simulink model "avg_inflow"  (R2022b)
settings: Solver=FixedStepDiscrete  StartTime=0  StopTime=duration  FixedStep=sample_time  RelTol=1e-3
values from neighbouring files (symbols this model uses):
  ParInflow_TUM =     [avg_inflow_params.mat]
libraries: simulink x10, dspstat3 x10
settings Model: Creator=Carlo_TUM  LastModifiedBy=Carlo_TUM
settings DataIOCC: LoadExternalInput=on  ReturnWorkspaceOutputs=off  ReturnWorkspaceOutputsName=off
settings OptimizationCC: DefaultParameterBehavior=Inlined  EnhancedBackFolding=on  PassReuseOutputArgsAs=Individual arguments  OptimizeBlockOrder=speed  DifferentSizesBufferReuse=on  OptimizationCustomize=off  EfficientTunableParamExpr=on
settings DebuggingCC: ParameterTunabilityLossMsg=error
settings SFSimCC: MATLABDynamicMemAlloc=off
settings RTWCC: Description=Embedded Coder  SystemTargetFile=ert.tlc  TemplateMakefile=ert_default_tmf
settings CodeAppCC: ForceParamTrailComments=on  IgnoreCustomStorageClasses=off  OperatorAnnotations=on  SimulinkDataObjDesc=on  SFDataObjDesc=on  InsertBlockDesc=on
settings ERTTargetCC: TargetLangStandard=C99 (ISO)  GenerateSampleERTMain=on  InlinedParameterPlacement=NonHierarchical  ERTCustomFileTemplate=example_file_process.tlc

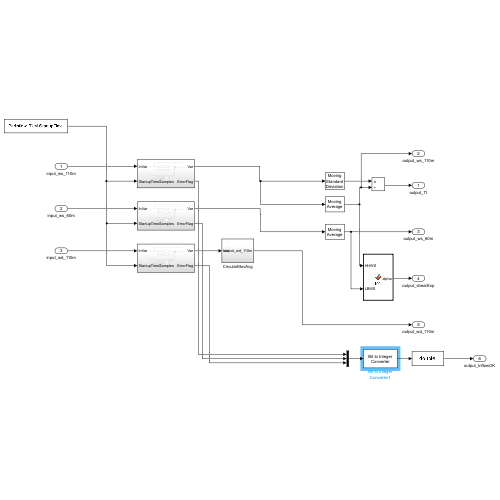
[thumbnail: Simulink's stored preview of the top-level diagram]
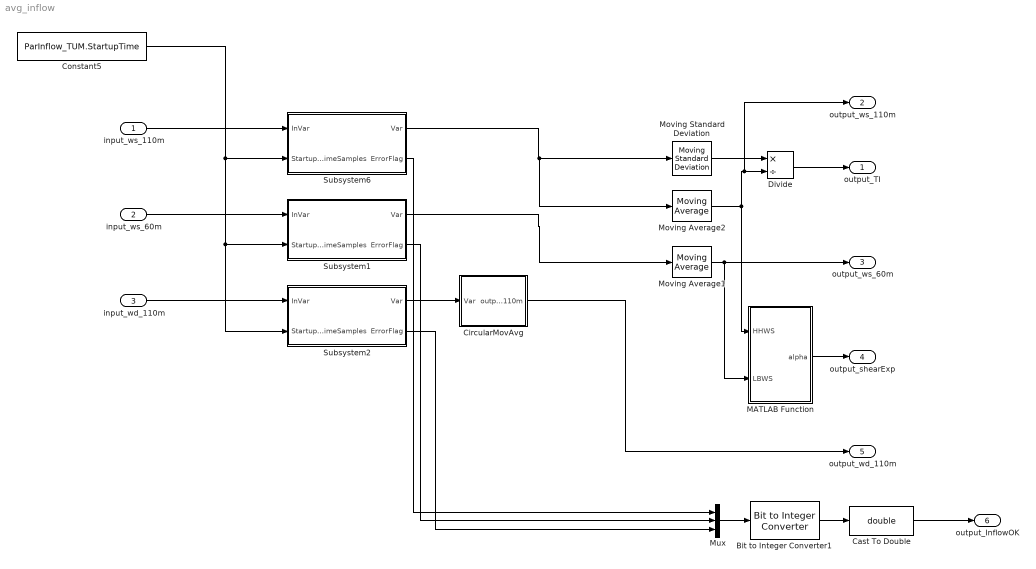
== system avg_inflow ==
  input_ws_110m : Inport  PortDimensions=1
  input_ws_60m : Inport  Port=2  PortDimensions=1
  input_wd_110m : Inport  Port=3  PortDimensions=1
  Bit to Integer Converter1 : simulink/Logic and Bit Operations/Bit to Integer Converter  nbits=3  bitOrder=MSB first  signedOutputValues=Unsigned  outDtype=Inherit via internal rule  outDtypeSigned=Inherit via internal rule
      settings: LibrarySourceBlock=|
      | commutil2/Bit to Integer
      | Converter
  Cast To Double : DataTypeConversion  OutDataTypeStr=double  SaturateOnIntegerOverflow=off  RndMeth=Floor
  CircularMovAvg : Subsystem
  Constant5 : Constant  Value=ParInflow_TUM.StartupTime
  Divide : Product  Inputs=*/
  MATLAB Function : MATLAB Function  TreatAsAtomicUnit=on
  Moving Average1 : dspstat3/Moving Average  Method=Sliding window  ForgettingFactorPort=off  SpecifyWindowLength=on  WindowLength=ParInflow_TUM.MovAvTI  OverlapLength=ParInflow_TUM.MovAvTI-1  AllowArbitraryInputLength=off  ForgettingFactor=0.9  SimulateUsing=Code generation
  Moving Average2 : dspstat3/Moving Average  Method=Sliding window  ForgettingFactorPort=off  SpecifyWindowLength=on  WindowLength=ParInflow_TUM.MovAvTI  OverlapLength=ParInflow_TUM.MovAvTI-1  AllowArbitraryInputLength=off  ForgettingFactor=0.9  SimulateUsing=Code generation
  Moving Standard Deviation : dspstat3/Moving Standard Deviation  Method=Sliding window  ForgettingFactorPort=off  SpecifyWindowLength=on  WindowLength=ParInflow_TUM.MovAvTI  OverlapLength=ParInflow_TUM.MovAvTI-1  AllowArbitraryInputLength=off  ForgettingFactor=0.9  SimulateUsing=Code generation
  Mux : Mux  Inputs=3
  Subsystem1 : Subsystem
  Subsystem2 : Subsystem
  Subsystem6 : Subsystem
  output_TI : Outport  VectorParamsAs1DForOutWhenUnconnected=off
  output_ws_110m : Outport  Port=2  VectorParamsAs1DForOutWhenUnconnected=off
  output_ws_60m : Outport  Port=3  VectorParamsAs1DForOutWhenUnconnected=off
  output_shearExp : Outport  Port=4  VectorParamsAs1DForOutWhenUnconnected=off
  output_wd_110m : Outport  Port=5  VectorParamsAs1DForOutWhenUnconnected=off
  output_InflowOK : Outport  Port=6  VectorParamsAs1DForOutWhenUnconnected=off
  wires:
  input_ws_110m/1 -> Subsystem6/1(InVar)
  input_ws_60m/1 -> Subsystem1/1(InVar)
  input_wd_110m/1 -> Subsystem2/1(InVar)
  Constant5/1 -> Subsystem2/2(StartupTimeSamples), Subsystem1/2(StartupTimeSamples), Subsystem6/2(StartupTimeSamples)
  Subsystem6/1(Var) -> Moving Average2/1, Moving Standard Deviation/1
  Subsystem1/1(Var) -> Moving Average1/1
  Moving Standard Deviation/1 -> Divide/1
  Moving Average2/1 -> MATLAB Function/1(HHWS), output_ws_110m/1, Divide/2
  Divide/1 -> output_TI/1
  Moving Average1/1 -> output_ws_60m/1, MATLAB Function/2(LBWS)
  MATLAB Function/1(alpha) -> output_shearExp/1
  Subsystem2/1(Var) -> CircularMovAvg/1(Var)
  CircularMovAvg/1(output_wd_110m) -> output_wd_110m/1
  Subsystem6/2(ErrorFlag) -> Mux/1
  Mux/1 -> Bit to Integer Converter1/1
  Subsystem2/2(ErrorFlag) -> Mux/3
  Subsystem1/2(ErrorFlag) -> Mux/2
  Bit to Integer Converter1/1 -> Cast To Double/1
  Cast To Double/1 -> output_InflowOK/1

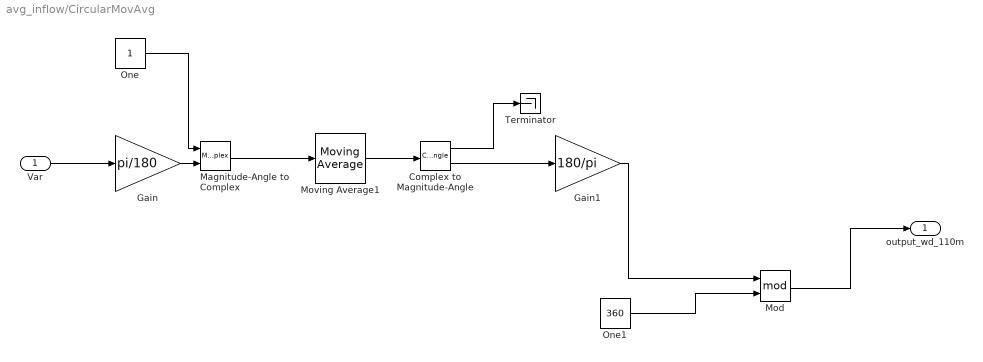
== system avg_inflow/CircularMovAvg ==
  Var : Inport
  Complex to Magnitude-Angle : ComplexToMagnitudeAngle
  Gain : Gain  Gain=pi/180
  Gain1 : Gain  Gain=180/pi
  Magnitude-Angle to Complex : MagnitudeAngleToComplex
  Mod : Math  Operator=mod  SignedPower=on
  Moving Average1 : dspstat3/Moving Average  Method=Sliding window  ForgettingFactorPort=off  SpecifyWindowLength=on  WindowLength=ParInflow_TUM.MovAvTI  OverlapLength=ParInflow_TUM.MovAvTI-1  AllowArbitraryInputLength=off  ForgettingFactor=0.9  SimulateUsing=Code generation
  One : Constant  OutDataTypeStr=Inherit: Inherit via back propagation
  One1 : Constant  Value=360  OutDataTypeStr=Inherit: Inherit via back propagation
  Terminator : Terminator
  output_wd_110m : Outport  VectorParamsAs1DForOutWhenUnconnected=off
  wires:
  Complex to Magnitude-Angle/2 -> Gain1/1
  Var/1 -> Gain/1
  One/1 -> Magnitude-Angle to Complex/1
  Gain/1 -> Magnitude-Angle to Complex/2
  Magnitude-Angle to Complex/1 -> Moving Average1/1
  Moving Average1/1 -> Complex to Magnitude-Angle/1
  Complex to Magnitude-Angle/1 -> Terminator/1
  Gain1/1 -> Mod/1
  One1/1 -> Mod/2
  Mod/1 -> output_wd_110m/1

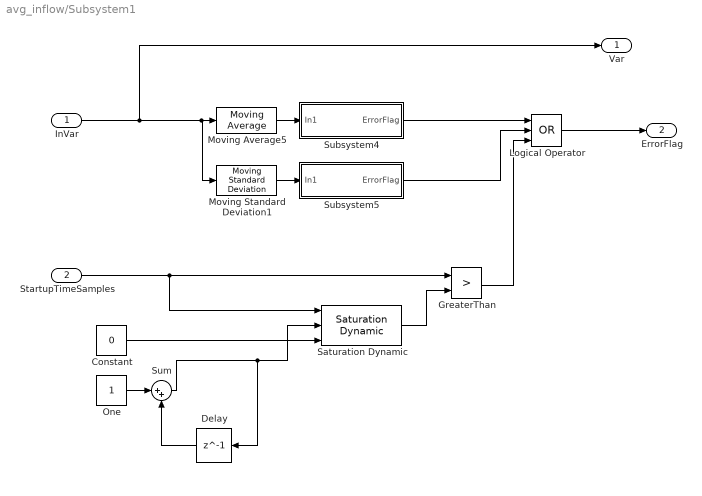
== system avg_inflow/Subsystem1 ==
  InVar : Inport
  StartupTimeSamples : Inport  Port=2
  Constant : Constant  Value=0
  Delay : Delay  DelayLength=1  InitialCondition=0
  GreaterThan : RelationalOperator  Operator=>  OutDataTypeStr=boolean  RndMeth=Simplest  InputSameDT=off
  Logical Operator : Logic  Operator=OR  Inputs=3  AllPortsSameDT=off  OutDataTypeStr=boolean
  Moving Average5 : dspstat3/Moving Average  Method=Sliding window  ForgettingFactorPort=off  SpecifyWindowLength=on  WindowLength=ParInflow_TUM.MovAvErrorCheck  OverlapLength=ParInflow_TUM.MovAvErrorCheck-1  AllowArbitraryInputLength=off  ForgettingFactor=0.9  SimulateUsing=Code generation
  Moving Standard Deviation1 : dspstat3/Moving Standard Deviation  Method=Sliding window  ForgettingFactorPort=off  SpecifyWindowLength=on  WindowLength=ParInflow_TUM.MovAvErrorCheck  OverlapLength=ParInflow_TUM.MovAvErrorCheck-1  AllowArbitraryInputLength=off  ForgettingFactor=0.9  SimulateUsing=Code generation
  One : Constant  OutDataTypeStr=Inherit: Inherit via back propagation
  Saturation Dynamic : simulink/Discontinuities/Saturation Dynamic  OutMin=[]  OutMax=[]  OutDataTypeStr=Inherit: Same as second input  OutDataType=fixdt(1, 16)  OutScaling=2^-10  DoSatur=off
  Subsystem4 : Subsystem
  Subsystem5 : Subsystem
  Sum : Sum  Inputs=|++
  Var : Outport  VectorParamsAs1DForOutWhenUnconnected=off
  ErrorFlag : Outport  Port=2  VectorParamsAs1DForOutWhenUnconnected=off
  wires:
  Saturation Dynamic/1 -> GreaterThan/2
  Constant/1 -> Saturation Dynamic/3
  GreaterThan/1 -> Logical Operator/3
  Delay/1 -> Sum/2
  One/1 -> Sum/1
  Sum/1 -> Saturation Dynamic/2, Delay/1
  StartupTimeSamples/1 -> GreaterThan/1, Saturation Dynamic/1
  Logical Operator/1 -> ErrorFlag/1
  Subsystem5/1(ErrorFlag) -> Logical Operator/2
  Moving Standard Deviation1/1 -> Subsystem5/1(In1)
  Subsystem4/1(ErrorFlag) -> Logical Operator/1
  Moving Average5/1 -> Subsystem4/1(In1)
  InVar/1 -> Moving Average5/1, Moving Standard Deviation1/1, Var/1

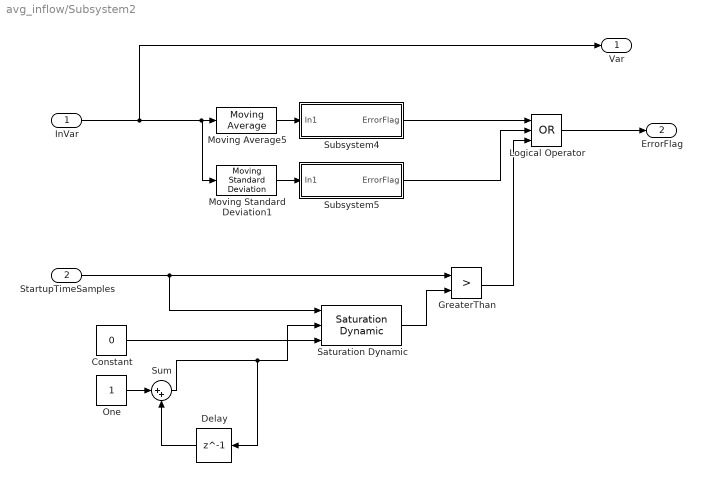
== system avg_inflow/Subsystem2 ==
  InVar : Inport
  StartupTimeSamples : Inport  Port=2
  Constant : Constant  Value=0
  Delay : Delay  DelayLength=1  InitialCondition=0
  GreaterThan : RelationalOperator  Operator=>  OutDataTypeStr=boolean  RndMeth=Simplest  InputSameDT=off
  Logical Operator : Logic  Operator=OR  Inputs=3  AllPortsSameDT=off  OutDataTypeStr=boolean
  Moving Average5 : dspstat3/Moving Average  Method=Sliding window  ForgettingFactorPort=off  SpecifyWindowLength=on  WindowLength=ParInflow_TUM.MovAvErrorCheck  OverlapLength=ParInflow_TUM.MovAvErrorCheck-1  AllowArbitraryInputLength=off  ForgettingFactor=0.9  SimulateUsing=Code generation
  Moving Standard Deviation1 : dspstat3/Moving Standard Deviation  Method=Sliding window  ForgettingFactorPort=off  SpecifyWindowLength=on  WindowLength=ParInflow_TUM.MovAvErrorCheck  OverlapLength=ParInflow_TUM.MovAvErrorCheck-1  AllowArbitraryInputLength=off  ForgettingFactor=0.9  SimulateUsing=Code generation
  One : Constant  OutDataTypeStr=Inherit: Inherit via back propagation
  Saturation Dynamic : simulink/Discontinuities/Saturation Dynamic  OutMin=[]  OutMax=[]  OutDataTypeStr=Inherit: Same as second input  OutDataType=fixdt(1, 16)  OutScaling=2^-10  DoSatur=off
  Subsystem4 : Subsystem
  Subsystem5 : Subsystem
  Sum : Sum  Inputs=|++
  Var : Outport  VectorParamsAs1DForOutWhenUnconnected=off
  ErrorFlag : Outport  Port=2  VectorParamsAs1DForOutWhenUnconnected=off
  wires:
  InVar/1 -> Var/1, Moving Standard Deviation1/1, Moving Average5/1
  Moving Average5/1 -> Subsystem4/1(In1)
  Subsystem4/1(ErrorFlag) -> Logical Operator/1
  Moving Standard Deviation1/1 -> Subsystem5/1(In1)
  Subsystem5/1(ErrorFlag) -> Logical Operator/2
  Logical Operator/1 -> ErrorFlag/1
  StartupTimeSamples/1 -> Saturation Dynamic/1, GreaterThan/1
  Sum/1 -> Delay/1, Saturation Dynamic/2
  One/1 -> Sum/1
  Delay/1 -> Sum/2
  GreaterThan/1 -> Logical Operator/3
  Constant/1 -> Saturation Dynamic/3
  Saturation Dynamic/1 -> GreaterThan/2

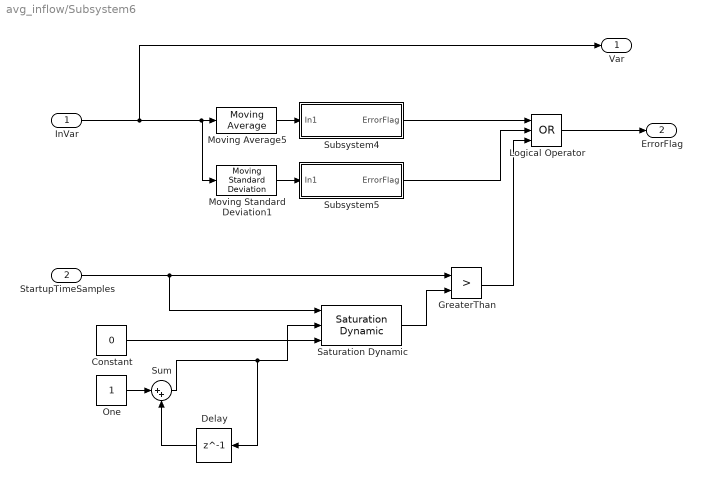
== system avg_inflow/Subsystem6 ==
  InVar : Inport
  StartupTimeSamples : Inport  Port=2
  Constant : Constant  Value=0
  Delay : Delay  DelayLength=1  InitialCondition=0
  GreaterThan : RelationalOperator  Operator=>  OutDataTypeStr=boolean  RndMeth=Simplest  InputSameDT=off
  Logical Operator : Logic  Operator=OR  Inputs=3  AllPortsSameDT=off  OutDataTypeStr=boolean
  Moving Average5 : dspstat3/Moving Average  Method=Sliding window  ForgettingFactorPort=off  SpecifyWindowLength=on  WindowLength=ParInflow_TUM.MovAvErrorCheck  OverlapLength=ParInflow_TUM.MovAvErrorCheck-1  AllowArbitraryInputLength=off  ForgettingFactor=0.9  SimulateUsing=Code generation
  Moving Standard Deviation1 : dspstat3/Moving Standard Deviation  Method=Sliding window  ForgettingFactorPort=off  SpecifyWindowLength=on  WindowLength=ParInflow_TUM.MovAvErrorCheck  OverlapLength=ParInflow_TUM.MovAvErrorCheck-1  AllowArbitraryInputLength=off  ForgettingFactor=0.9  SimulateUsing=Code generation
  One : Constant  OutDataTypeStr=Inherit: Inherit via back propagation
  Saturation Dynamic : simulink/Discontinuities/Saturation Dynamic  OutMin=[]  OutMax=[]  OutDataTypeStr=Inherit: Same as second input  OutDataType=fixdt(1, 16)  OutScaling=2^-10  DoSatur=off
  Subsystem4 : Subsystem
  Subsystem5 : Subsystem
  Sum : Sum  Inputs=|++
  Var : Outport  VectorParamsAs1DForOutWhenUnconnected=off
  ErrorFlag : Outport  Port=2  VectorParamsAs1DForOutWhenUnconnected=off
  wires:
  InVar/1 -> Var/1, Moving Standard Deviation1/1, Moving Average5/1
  Moving Average5/1 -> Subsystem4/1(In1)
  Subsystem4/1(ErrorFlag) -> Logical Operator/1
  Moving Standard Deviation1/1 -> Subsystem5/1(In1)
  Subsystem5/1(ErrorFlag) -> Logical Operator/2
  Logical Operator/1 -> ErrorFlag/1
  StartupTimeSamples/1 -> Saturation Dynamic/1, GreaterThan/1
  Sum/1 -> Delay/1, Saturation Dynamic/2
  One/1 -> Sum/1
  Delay/1 -> Sum/2
  GreaterThan/1 -> Logical Operator/3
  Constant/1 -> Saturation Dynamic/3
  Saturation Dynamic/1 -> GreaterThan/2

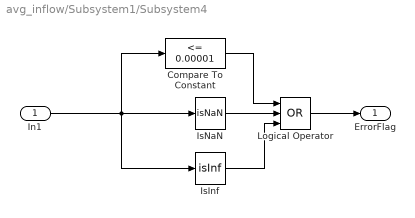
== system avg_inflow/Subsystem1/Subsystem4 ==
  In1 : Inport
  Compare To Constant : simulink/Logic and Bit Operations/Compare To Constant  relop=<=  const=0.00001  OutDataTypeStr=boolean
  IsInf : RelationalOperator  Operator=isInf  OutDataTypeStr=boolean  RndMeth=Simplest  InputSameDT=off
  IsNaN : RelationalOperator  Operator=isNaN  OutDataTypeStr=boolean  RndMeth=Simplest  InputSameDT=off
  Logical Operator : Logic  Operator=OR  Inputs=3  AllPortsSameDT=off  OutDataTypeStr=boolean
  ErrorFlag : Outport  VectorParamsAs1DForOutWhenUnconnected=off
  wires:
  IsNaN/1 -> Logical Operator/2
  In1/1 -> Compare To Constant/1, IsNaN/1, IsInf/1
  IsInf/1 -> Logical Operator/3
  Logical Operator/1 -> ErrorFlag/1
  Compare To Constant/1 -> Logical Operator/1

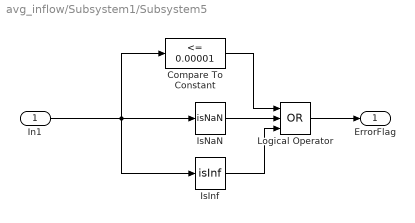
== system avg_inflow/Subsystem1/Subsystem5 ==
  In1 : Inport
  Compare To Constant : simulink/Logic and Bit Operations/Compare To Constant  relop=<=  const=0.00001  OutDataTypeStr=boolean
  IsInf : RelationalOperator  Operator=isInf  OutDataTypeStr=boolean  RndMeth=Simplest  InputSameDT=off
  IsNaN : RelationalOperator  Operator=isNaN  OutDataTypeStr=boolean  RndMeth=Simplest  InputSameDT=off
  Logical Operator : Logic  Operator=OR  Inputs=3  AllPortsSameDT=off  OutDataTypeStr=boolean
  ErrorFlag : Outport  VectorParamsAs1DForOutWhenUnconnected=off
  wires:
  Compare To Constant/1 -> Logical Operator/1
  Logical Operator/1 -> ErrorFlag/1
  IsInf/1 -> Logical Operator/3
  In1/1 -> Compare To Constant/1, IsInf/1, IsNaN/1
  IsNaN/1 -> Logical Operator/2

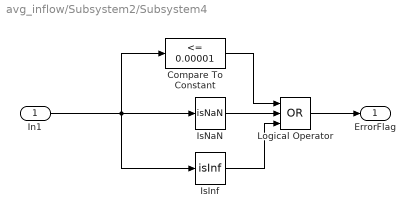
== system avg_inflow/Subsystem2/Subsystem4 ==
  In1 : Inport
  Compare To Constant : simulink/Logic and Bit Operations/Compare To Constant  relop=<=  const=0.00001  OutDataTypeStr=boolean
  IsInf : RelationalOperator  Operator=isInf  OutDataTypeStr=boolean  RndMeth=Simplest  InputSameDT=off
  IsNaN : RelationalOperator  Operator=isNaN  OutDataTypeStr=boolean  RndMeth=Simplest  InputSameDT=off
  Logical Operator : Logic  Operator=OR  Inputs=3  AllPortsSameDT=off  OutDataTypeStr=boolean
  ErrorFlag : Outport  VectorParamsAs1DForOutWhenUnconnected=off
  wires:
  Compare To Constant/1 -> Logical Operator/1
  Logical Operator/1 -> ErrorFlag/1
  IsInf/1 -> Logical Operator/3
  In1/1 -> IsInf/1, IsNaN/1, Compare To Constant/1
  IsNaN/1 -> Logical Operator/2

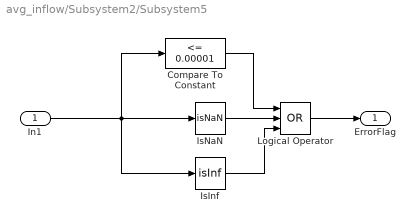
== system avg_inflow/Subsystem2/Subsystem5 ==
  In1 : Inport
  Compare To Constant : simulink/Logic and Bit Operations/Compare To Constant  relop=<=  const=0.00001  OutDataTypeStr=boolean
  IsInf : RelationalOperator  Operator=isInf  OutDataTypeStr=boolean  RndMeth=Simplest  InputSameDT=off
  IsNaN : RelationalOperator  Operator=isNaN  OutDataTypeStr=boolean  RndMeth=Simplest  InputSameDT=off
  Logical Operator : Logic  Operator=OR  Inputs=3  AllPortsSameDT=off  OutDataTypeStr=boolean
  ErrorFlag : Outport  VectorParamsAs1DForOutWhenUnconnected=off
  wires:
  IsNaN/1 -> Logical Operator/2
  In1/1 -> IsNaN/1, IsInf/1, Compare To Constant/1
  IsInf/1 -> Logical Operator/3
  Logical Operator/1 -> ErrorFlag/1
  Compare To Constant/1 -> Logical Operator/1

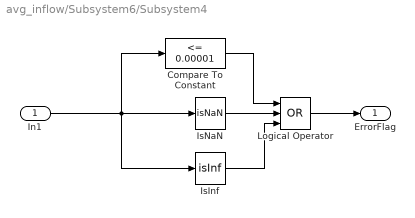
== system avg_inflow/Subsystem6/Subsystem4 ==
  In1 : Inport
  Compare To Constant : simulink/Logic and Bit Operations/Compare To Constant  relop=<=  const=0.00001  OutDataTypeStr=boolean
  IsInf : RelationalOperator  Operator=isInf  OutDataTypeStr=boolean  RndMeth=Simplest  InputSameDT=off
  IsNaN : RelationalOperator  Operator=isNaN  OutDataTypeStr=boolean  RndMeth=Simplest  InputSameDT=off
  Logical Operator : Logic  Operator=OR  Inputs=3  AllPortsSameDT=off  OutDataTypeStr=boolean
  ErrorFlag : Outport  VectorParamsAs1DForOutWhenUnconnected=off
  wires:
  Compare To Constant/1 -> Logical Operator/1
  Logical Operator/1 -> ErrorFlag/1
  IsInf/1 -> Logical Operator/3
  In1/1 -> IsInf/1, IsNaN/1, Compare To Constant/1
  IsNaN/1 -> Logical Operator/2

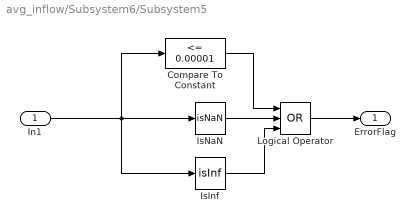
== system avg_inflow/Subsystem6/Subsystem5 ==
  In1 : Inport
  Compare To Constant : simulink/Logic and Bit Operations/Compare To Constant  relop=<=  const=0.00001  OutDataTypeStr=boolean
  IsInf : RelationalOperator  Operator=isInf  OutDataTypeStr=boolean  RndMeth=Simplest  InputSameDT=off
  IsNaN : RelationalOperator  Operator=isNaN  OutDataTypeStr=boolean  RndMeth=Simplest  InputSameDT=off
  Logical Operator : Logic  Operator=OR  Inputs=3  AllPortsSameDT=off  OutDataTypeStr=boolean
  ErrorFlag : Outport  VectorParamsAs1DForOutWhenUnconnected=off
  wires:
  IsNaN/1 -> Logical Operator/2
  In1/1 -> IsNaN/1, IsInf/1, Compare To Constant/1
  IsInf/1 -> Logical Operator/3
  Logical Operator/1 -> ErrorFlag/1
  Compare To Constant/1 -> Logical Operator/1

== matlab function avg_inflow/MATLAB Function ==
  data: HHWS input; alpha output; LBWS input
function alpha = fcn(HHWS, LBWS)

alpha = (log(HHWS) - log(LBWS))./(log(110) - log(60)); %% CRS: this needs to be modified with the real heights
